simulink model "Twostage_TVC6DOF_sim"  (R2023b)
settings: Solver=VariableStepAuto  StartTime=0.0  StopTime=7  RelTol=1e-3
values from neighbouring files (symbols this model uses):
  g = 9.81    [TVC6DOF.m]
  ignition_delay_mc = ignition_delay_n+randn*ignition_delay_v    [TVC6DOF.m]
  Ix2_mc = Ix2_n+randn*Ix2_v    [TVC6DOF.m]
  Ix_mc = Ix_n+randn*Ix_v    [TVC6DOF.m]
  Iy2_mc = Iy2_n+randn*Iy2_v    [TVC6DOF.m]
  Iy_mc = Iy_n+randn*Iy_v    [TVC6DOF.m]
  Iz2_mc = Iz2_n+randn*Iz2_v    [TVC6DOF.m]
  Iz_mc = Iz_n+randn*Iz_v    [TVC6DOF.m]
  l2_mc = l2_n+randn*l2_v    [TVC6DOF.m]
  l_mc = l_n+randn*l_v    [TVC6DOF.m]
  m2_dry_mc = m2_dry_n+randn*m2_dry_v    [TVC6DOF.m]
  m_dry_mc = m_dry_n+randn*m_dry_v    [TVC6DOF.m]
  mis_y_mc = randn*mis_y_v    [TVC6DOF.m]
  mis_z_mc = randn*mis_z_v    [TVC6DOF.m]
  servo_delay_mc = servo_delay_n+randn*servo_delay_v    [TVC6DOF.m]
  twostage_delay_n = 1.5    [TVC6DOF.m]
undefined symbols (not defined in the file or in its folder): sigbuilder_block
settings Model: Creator=govindchari  LastModifiedBy=AISL
settings SolverCC: AlgebraicLoopSolver=TrustRegion
settings DebuggingCC: UnconnectedInputMsg=warning  UnconnectedOutputMsg=warning  UnconnectedLineMsg=warning
settings ModelReferenceCC: EnableRefExpFcnMdlSchedulingChecks=on
settings RTWCC: DLArmComputeVersion=19.05

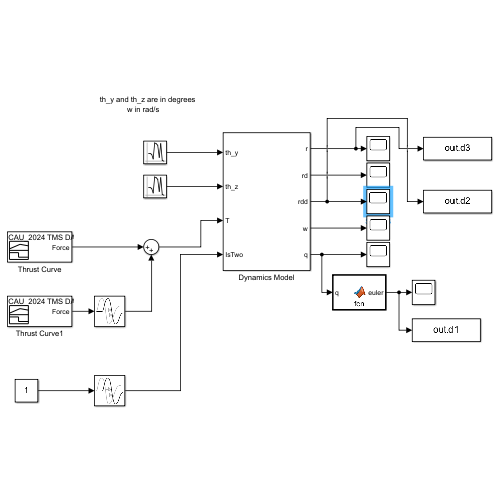
[thumbnail: Simulink's stored preview of the top-level diagram]
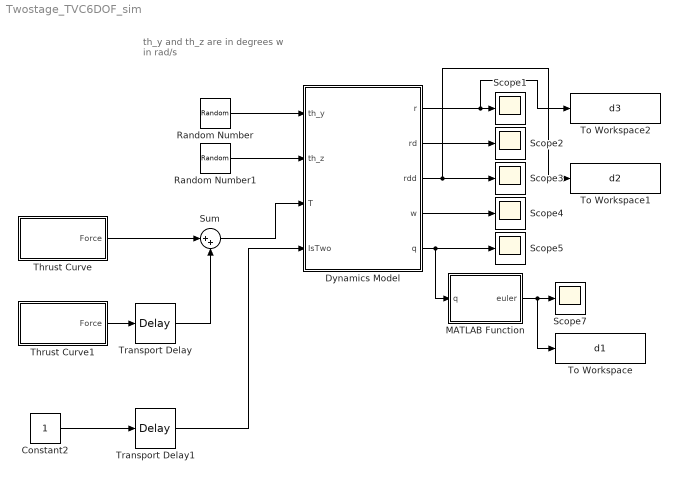
== system Twostage_TVC6DOF_sim ==
  note: th_y and th_z are in degrees
      |              w in rad/s
  Constant2 : Constant
  Dynamics Model : Subsystem
  MATLAB Function : MATLAB Function  TreatAsAtomicUnit=on
  Random Number : RandomNumber  Variance=0.1  SampleTime=0.001
  Random Number1 : RandomNumber  Variance=0.1  SampleTime=0.001
  Scope{1..5,7} (6 alike) : Scope
  Sum : Sum  Inputs=|++
  Thrust Curve : Subsystem  Tag=STV Subsys  LoadFcn=sigbuilder_block('load');  StartFcn=sigbuilder_block('start');  StopFcn=sigbuilder_block('stop');  ClipboardFcn=sigbuilder_block('clipboard');  mask(Sigbuilder block){tuvar=[0:10]}
      mask help: Simulink:masks:SigbuilderBlock_MD
      mask init:
      | if ~strcmp(get_param(bdroot(gcbh),'SimulationStatus'),'stopped') tuvar = sigbuilder_block('maskInit'); end
      settings: CopyFcn=sigbuilder_block('copy');  DeleteFcn=sigbuilder_block('delete');  ModelCloseFcn=sigbuilder_block('modelClose');  PreSaveFcn=sigbuilder_block('preSave');  PauseFcn=sigbuilder_block('pause');  ContinueFcn=sigbuilder_block('continue');  NameChangeFcn=sigbuilder_block('namechange');  OpenFcn=sigbuilder_block('open',[1201.5 112.5 712.5 317.25 ]);  CloseFcn=sigbuilder_block('close');
      mask Display: plot(0, 0, 100, 100,[2, 2, 32, 32, 2], [68, 8, 8, 68, 68],[32, 2], [38, 38], [32, 19, 2],[53, 60, 44], [32, 17, 17, 2],[16, 16, 31, 31]);txt = getActiveGroup(gcbh);text(2, 100, txt,'verticalAlignment', 'top');
  Thrust Curve1 : Subsystem  Tag=STV Subsys  LoadFcn=sigbuilder_block('load');  StartFcn=sigbuilder_block('start');  StopFcn=sigbuilder_block('stop');  ClipboardFcn=sigbuilder_block('clipboard');  mask(Sigbuilder block){tuvar=[0:10]}
      mask help: Simulink:masks:SigbuilderBlock_MD
      mask init:
      | if ~strcmp(get_param(bdroot(gcbh),'SimulationStatus'),'stopped') tuvar = sigbuilder_block('maskInit'); end
      settings: CopyFcn=sigbuilder_block('copy');  DeleteFcn=sigbuilder_block('delete');  ModelCloseFcn=sigbuilder_block('modelClose');  PreSaveFcn=sigbuilder_block('preSave');  PauseFcn=sigbuilder_block('pause');  ContinueFcn=sigbuilder_block('continue');  NameChangeFcn=sigbuilder_block('namechange');  OpenFcn=sigbuilder_block('open',[380.25 420 924.75 358.5 ]);  CloseFcn=sigbuilder_block('close');
      mask Display: plot(0, 0, 100, 100,[2, 2, 32, 32, 2], [68, 8, 8, 68, 68],[32, 2], [38, 38], [32, 19, 2],[53, 60, 44], [32, 17, 17, 2],[16, 16, 31, 31]);txt = getActiveGroup(gcbh);text(2, 100, txt,'verticalAlignment', 'top');
  To Workspace : ToWorkspace  VariableName=d1  SaveFormat=Timeseries  SampleTime=-1
  To Workspace1 : ToWorkspace  VariableName=d2  SaveFormat=Timeseries  SampleTime=-1
  To Workspace2 : ToWorkspace  VariableName=d3  SaveFormat=Timeseries  SampleTime=-1
  Transport Delay : TransportDelay  DelayTime=ignition_delay_mc+servo_delay_mc+twostage_delay_n
  Transport Delay1 : TransportDelay  DelayTime=servo_delay_mc+twostage_delay_n
  wires:
  Dynamics Model/1(r) -> To Workspace2/1, Scope1/1
  Dynamics Model/2(rd) -> Scope2/1
  Dynamics Model/5(q) -> MATLAB Function/1(q), Scope5/1
  Dynamics Model/4(w) -> Scope4/1
  Dynamics Model/3(rdd) -> Scope3/1, To Workspace1/1
  Random Number/1 -> Dynamics Model/1(th_y)
  Random Number1/1 -> Dynamics Model/2(th_z)
  Sum/1 -> Dynamics Model/3(T)
  Thrust Curve/1(Force) -> Sum/1
  Thrust Curve1/1(Force) -> Transport Delay/1
  Transport Delay/1 -> Sum/2
  Constant2/1 -> Transport Delay1/1
  Transport Delay1/1 -> Dynamics Model/4(IsTwo)
  MATLAB Function/1(euler) -> To Workspace/1, Scope7/1

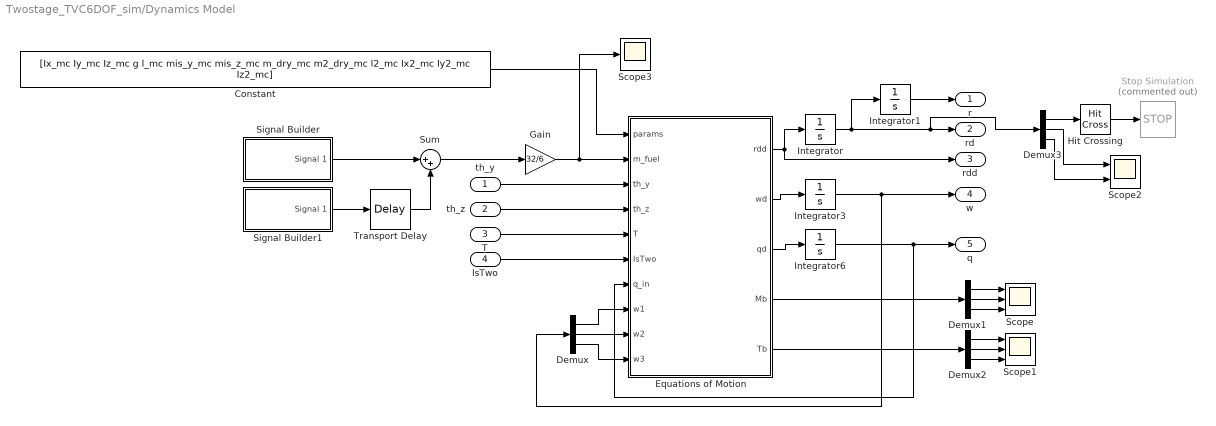
== system Twostage_TVC6DOF_sim/Dynamics Model ==
  th_y : Inport
  th_z : Inport  Port=2
  T : Inport  Port=3
  IsTwo : Inport  Port=4
  Constant : Constant  Value=[Ix_mc Iy_mc Iz_mc g l_mc mis_y_mc mis_z_mc m_dry_mc m2_dry_mc l2_mc Ix2_mc Iy2_mc Iz2_mc]
  Demux{,1..3} (4 alike) : Demux  Outputs=3
  Equations of Motion : MATLAB Function  TreatAsAtomicUnit=on
  Gain : Gain  Gain=32/6
  Hit Crossing : HitCross  HitCrossingOffset=0.01  HitCrossingDirection=falling
  Integrator : Integrator  InitialCondition=[0 0 0]
  Integrator1 : Integrator  InitialCondition=[0 0 0]
  Integrator3 : Integrator  InitialCondition=[0 0 0]
  Integrator6 : Integrator  InitialCondition=[1 0 0 0]
  Scope : Scope  NumInputPorts=3
  Scope1 : Scope  NumInputPorts=3
  Scope2 : Scope  NumInputPorts=2
  Scope3 : Scope
  Signal Builder : Subsystem  Tag=STV Subsys  LoadFcn=sigbuilder_block('load');  StartFcn=sigbuilder_block('start');  StopFcn=sigbuilder_block('stop');  ClipboardFcn=sigbuilder_block('clipboard');  mask(Sigbuilder block){tuvar=[0:10]}
      mask help: Simulink:masks:SigbuilderBlock_MD
      mask init:
      | if ~strcmp(get_param(bdroot(gcbh),'SimulationStatus'),'stopped') tuvar = sigbuilder_block('maskInit'); end
      settings: CopyFcn=sigbuilder_block('copy');  DeleteFcn=sigbuilder_block('delete');  ModelCloseFcn=sigbuilder_block('modelClose');  PreSaveFcn=sigbuilder_block('preSave');  PauseFcn=sigbuilder_block('pause');  ContinueFcn=sigbuilder_block('continue');  NameChangeFcn=sigbuilder_block('namechange');  OpenFcn=sigbuilder_block('open',[1949.25 96 550.5 400.5 ]);  CloseFcn=sigbuilder_block('close');
      mask Display: plot(0, 0, 100, 100,[2, 2, 32, 32, 2], [68, 8, 8, 68, 68],[32, 2], [38, 38], [32, 19, 2],[53, 60, 44], [32, 17, 17, 2],[16, 16, 31, 31]);txt = getActiveGroup(gcbh);text(2, 100, txt,'verticalAlignment', 'top');
  Signal Builder1 : Subsystem  Tag=STV Subsys  LoadFcn=sigbuilder_block('load');  StartFcn=sigbuilder_block('start');  StopFcn=sigbuilder_block('stop');  ClipboardFcn=sigbuilder_block('clipboard');  mask(Sigbuilder block){tuvar=[0:10]}
      mask help: Simulink:masks:SigbuilderBlock_MD
      mask init:
      | if ~strcmp(get_param(bdroot(gcbh),'SimulationStatus'),'stopped') tuvar = sigbuilder_block('maskInit'); end
      settings: CopyFcn=sigbuilder_block('copy');  DeleteFcn=sigbuilder_block('delete');  ModelCloseFcn=sigbuilder_block('modelClose');  PreSaveFcn=sigbuilder_block('preSave');  PauseFcn=sigbuilder_block('pause');  ContinueFcn=sigbuilder_block('continue');  NameChangeFcn=sigbuilder_block('namechange');  OpenFcn=sigbuilder_block('open',[1949.25 96 550.5 400.5 ]);  CloseFcn=sigbuilder_block('close');
      mask Display: plot(0, 0, 100, 100,[2, 2, 32, 32, 2], [68, 8, 8, 68, 68],[32, 2], [38, 38], [32, 19, 2],[53, 60, 44], [32, 17, 17, 2],[16, 16, 31, 31]);txt = getActiveGroup(gcbh);text(2, 100, txt,'verticalAlignment', 'top');
  Stop Simulation : Stop  Commented=on
  Sum : Sum  Inputs=|++
  Transport Delay : TransportDelay  DelayTime=ignition_delay_mc+servo_delay_mc+twostage_delay_n  InitialOutput=60
  r : Outport
  rd : Outport  Port=2
  rdd : Outport  Port=3
  w : Outport  Port=4
  q : Outport  Port=5
  wires:
  Constant/1 -> Equations of Motion/1(params)
  Equations of Motion/3(qd) -> Integrator6/1
  Equations of Motion/2(wd) -> Integrator3/1
  Equations of Motion/1(rdd) -> Integrator/1, rdd/1
  T/1 -> Equations of Motion/5(T)
  Integrator/1 -> Integrator1/1, Demux3/1, rd/1
  Integrator1/1 -> r/1
  Demux/1 -> Equations of Motion/8(w1)
  Demux/2 -> Equations of Motion/9(w2)
  Demux/3 -> Equations of Motion/10(w3)
  Integrator6/1 -> Equations of Motion/7(q_in), q/1
  Integrator3/1 -> Demux/1, w/1
  Equations of Motion/4(Mb) -> Demux1/1
  Equations of Motion/5(Tb) -> Demux2/1
  Demux1/1 -> Scope/1
  Demux1/2 -> Scope/2
  Demux1/3 -> Scope/3
  Demux2/1 -> Scope1/1
  Demux2/2 -> Scope1/2
  Demux2/3 -> Scope1/3
  Demux3/1 -> Hit Crossing/1
  Hit Crossing/1 -> Stop Simulation/1
  Demux3/2 -> Scope2/1
  Demux3/3 -> Scope2/2
  th_z/1 -> Equations of Motion/4(th_z)
  th_y/1 -> Equations of Motion/3(th_y)
  Gain/1 -> Scope3/1, Equations of Motion/2(m_fuel)
  IsTwo/1 -> Equations of Motion/6(IsTwo)
  Signal Builder/1(Signal 1) -> Sum/1
  Sum/1 -> Gain/1
  Signal Builder1/1(Signal 1) -> Transport Delay/1
  Transport Delay/1 -> Sum/2

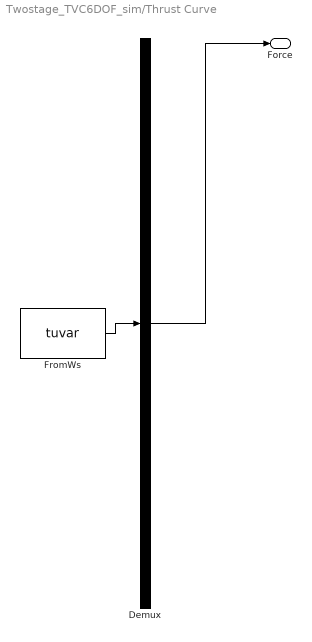
== system Twostage_TVC6DOF_sim/Thrust Curve ==
  Demux : Demux  Tag=STV Demux  Outputs=1
      settings: DisplayOption=none
  FromWs : FromWorkspace  Tag=STV FromWs  VariableName=tuvar
      SigBuilderData=|
      | common.afterFinalStr = 'Extrapolate'
      | common.sampleTime = 0
      | dataSet.timeRange = [0 7]
      | dataSet.name = 'CAU_2024 TMS DATA_0525'
      | sbobj.Groups.Name = 'CAU_2024 TMS DATA_0525'
      | sbobj.Groups.Signals.Name = 'Force'
      | sbobj.Groups.Signals.XData = [0 0.06 0.13 0.2 0.27 0.34 0.41 0.47 0.54 0.61 0.68 0.75 0.82 0.88 0.95 1.02 1.09 1.16 1.23 1.3 1.36 1.43 1.5 1.56 1.63 1.7 1.77 1.84 1.9 1.97 2.04 2.11 2.17 2.24 2.31 2.38 2.44 2.51 2.58 7]
      | sbobj.Groups.Signals.YData = [20.593965 10.591182 23.339827 42.6589275 69.7252815 112.4822755 170.047311 259.7781585 451.890432 466.3340375 466.432104 467.412769 479.371316 469.346269 340.094622 265.6621485 130.9187775 44.8163905 20.986231 10.4931155 2.2555295 1.569064 0.0980665 0 1.4709975 0.2941995 0.784532 0.196133 0 0 0.392266 0 1.6671305 1.176798 0 1.2748645 0.2941995 0 1.372931 1.372931]
      | sbobj.Groups.TimeRange = [0 7]
  Force : Outport  Tag=STV Outport
  wires:
  Demux/1 -> Force/1
  FromWs/1 -> Demux/1

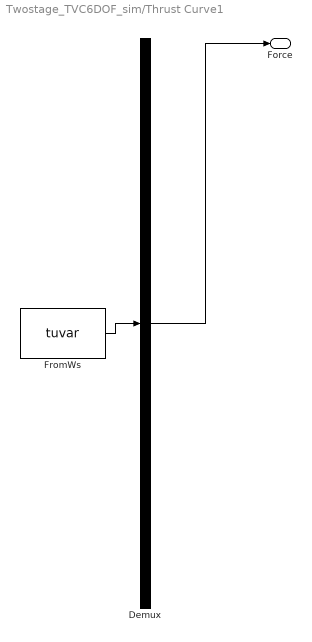
== system Twostage_TVC6DOF_sim/Thrust Curve1 ==
  Demux : Demux  Tag=STV Demux  Outputs=1
      settings: DisplayOption=none
  FromWs : FromWorkspace  Tag=STV FromWs  VariableName=tuvar
      SigBuilderData=|
      | common.afterFinalStr = 'Extrapolate'
      | common.sampleTime = 0
      | dataSet(1).timeRange = [0 2.58]
      | dataSet(1).name = 'CAU_2024 TMS DATA_0525'
      | dataSet(2).timeRange = [0 7]
      | dataSet(2).name = 'CAU_2024 TMS DATA_1'
      | dataSet(3).timeRange = [0 7]
      | dataSet(3).name = 'CAU_2024 TMS DATA_2'
      | sbobj.Groups(1).Name = 'CAU_2024 TMS DATA_0525'
      | sbobj.Groups(1).Signals.Name = 'Force'
      | sbobj.Groups(1).Signals.XData = [0 0.06 0.13 0.2 0.27 0.34 0.41 0.47 0.54 0.61 0.68 0.75 0.82 0.88 0.95 1.02 1.09 1.16 1.23 1.3 1.36 1.43 1.5 1.56 1.63 1.7 1.77 1.84 1.9 1.97 2.04 2.11 2.17 2.24 2.31 2.38 2.44 2.51 2.58]
      | sbobj.Groups(1).Signals.YData = [20.593965 10.591182 23.339827 42.6589275 69.7252815 112.4822755 170.047311 259.7781585 451.890432 466.3340375 466.432104 467.412769 479.371316 469.346269 340.094622 265.6621485 130.9187775 44.8163905 20.986231 10.4931155 2.2555295 1.569064 0.0980665 0 1.4709975 0.2941995 0.784532 0.196133 0 0 0.392266 0 1.6671305 1.176798 0 1.2748645 0.2941995 0 1.372931]
      | sbobj.Groups(1).TimeRange = [0 2.58]
      | sbobj.Groups(2).Name = 'CAU_2024 TMS DATA_1'
      | sbobj.Groups(2).Signals.Name = 'Force'
      | sbobj.Groups(2).Signals.XData = [0 0.06 0.13 0.2 0.27 0.34 0.41 0.47 0.54 0.61 0.68 0.75 0.82 0.88 0.95 1.02 1.09 1.16 1.23 1.3 1.36 1.43 1.5 1.56 1.63 1.7 1.77 1.84 1.9 1.97 2.04 2.11 2.17 2.24 2.31 2.38 2.44 2.51 2.58 7]
      | sbobj.Groups(2).Signals.YData = [20.593965 10.591182 23.339827 42.6589275 69.7252815 112.4822755 170.047311 259.7781585 451.890432 466.3340375 466.432104 467.412769 479.371316 469.346269 340.094622 265.6621485 130.9187775 44.8163905 20.986231 10.4931155 2.2555295 1.569064 0.0980665 0 1.4709975 0.2941995 0.784532 0.196133 0 0 0.392266 0 1.6671305 1.176798 0 1.2748645 0.2941995 0 1.372931 1.372931]
      | sbobj.Groups(2).TimeRange = [0 7]
      | sbobj.Groups(3).Name = 'CAU_2024 TMS DATA_2'
      | sbobj.Groups(3).Signals.Name = 'Force'
      | sbobj.Groups(3).Signals.XData = [0 2 2.07 2.14 2.21 2.27 2.34 2.41 2.48 2.54 2.61 2.68 2.75 2.82 2.89 2.95 3.02 3.09 3.16 3.23 3.3 3.36 3.43 3.5 3.57 3.64 3.71 3.78 3.84 3.91 3.98 4.04 4.11 4.18 4.25 4.32 4.38 4.45 4.52 4.59 4.65 4.72 4.79 4.86 4.92 4.99 5.06 7]
      | sbobj.Groups(3).Signals.YData = [0 0 0 0 0 0.392266 0 0.392266 20.593965 10.591182 23.339827 42.6589275 69.7252815 112.4822755 170.047311 259.7781585 451.890432 466.3340375 466.432104 467.412769 479.371316 469.346269 340.094622 265.6621485 130.9187775 44.8163905 20.986231 10.4931155 2.2555295 1.569064 0.0980665 0 1.4709975 0.2941995 0.784532 0.196133 0 0 0.392266 0 1.6671305 1.176798 0 1.2748645 0.2941995 0 1.372931 1.372931]
      | sbobj.Groups(3).TimeRange = [0 7]
  Force : Outport  Tag=STV Outport
  wires:
  Demux/1 -> Force/1
  FromWs/1 -> Demux/1

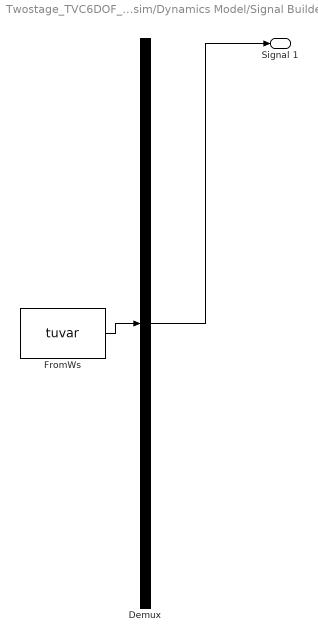
== system Twostage_TVC6DOF_sim/Dynamics Model/Signal Builder ==
  Demux : Demux  Tag=STV Demux  Outputs=1
      settings: DisplayOption=none
  FromWs : FromWorkspace  Tag=STV FromWs  VariableName=tuvar
      SigBuilderData=|
      | common.afterFinalStr = 'Extrapolate'
      | common.sampleTime = 0
      | dataSet.timeRange = [0 10]
      | dataSet.name = 'Group 1'
      | sbobj.Groups.Name = 'Group 1'
      | sbobj.Groups.Signals.Name = 'Signal 1'
      | sbobj.Groups.Signals.XData = [0 0.148 0.228 0.294 0.419 0.477 0.52 0.593 0.628 0.755 0.837 1 1.123 1.152 1.163 1.286 1.455 1.61 1.694 1.71 1.72 1.75 3.404 3.404 3.45 9.8 10]
      | sbobj.Groups.Signals.YData = [60 59.3164 58.3541 57.2108 54.0771 52.3818 51.2397 49.4767 47.3744 43.9685 40.4849 37.3989 33.5 32.9674 32.026 27.8823 24.0514 19.5 14.8632 10.4455 4.68731 0.51289 0.215344 0.0947253 0 0 0]
  Signal 1 : Outport  Tag=STV Outport
  wires:
  Demux/1 -> Signal 1/1
  FromWs/1 -> Demux/1

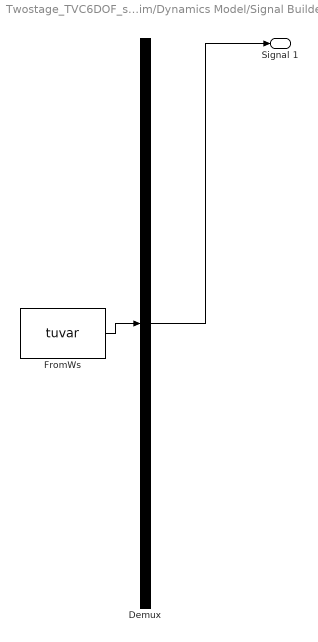
== system Twostage_TVC6DOF_sim/Dynamics Model/Signal Builder1 ==
  Demux : Demux  Tag=STV Demux  Outputs=1
      settings: DisplayOption=none
  FromWs : FromWorkspace  Tag=STV FromWs  VariableName=tuvar
      SigBuilderData=|
      | common.afterFinalStr = 'Extrapolate'
      | common.sampleTime = 0
      | dataSet.timeRange = [0 10]
      | dataSet.name = 'Group 1'
      | sbobj.Groups.Name = 'Group 1'
      | sbobj.Groups.Signals.Name = 'Signal 1'
      | sbobj.Groups.Signals.XData = [0 0.148 0.228 0.294 0.419 0.477 0.52 0.593 0.628 0.755 0.837 1 1.123 1.152 1.163 1.286 1.455 1.61 1.694 1.71 1.72 1.75 3.404 3.404 3.45 9.8 10]
      | sbobj.Groups.Signals.YData = [60 59.3164 58.3541 57.2108 54.0771 52.3818 51.2397 49.4767 47.3744 43.9685 40.4849 37.3989 33.5 32.9674 32.026 27.8823 24.0514 19.5 14.8632 10.4455 4.68731 0.51289 0.215344 0.0947253 0 0 0]
  Signal 1 : Outport  Tag=STV Outport
  wires:
  Demux/1 -> Signal 1/1
  FromWs/1 -> Demux/1

== matlab function Twostage_TVC6DOF_sim/MATLAB Function ==
  data: q input; euler output
function euler = fcn(q)
euler=[1,1,1];
euler = quat2eul(q');

== matlab function Twostage_TVC6DOF_sim/Dynamics Model/Equations of Motion ==
  data: params input; m_fuel input; th_y input; rdd output; th_z input; T input; IsTwo input; q_in input; wd output; qd output; w1 input; w2 input; w3 input; Mb output; Tb output
function [rdd,wd,qd,Mb,Tb] = EOM(params,m_fuel,th_y,th_z,T,IsTwo, q_in,w1,w2,w3)
Ix=params(1);
Iy=params(2);
Iz=params(3);
g=params(4);
l=params(5);
mis_y=params(6);
mis_z=params(7);
m_dry=params(8);
m2_dry=params(9);
l2=params(10);
Ix2=params(11);
Iy2=params(12);
Iz2=params(13);

if(IsTwo==0)
    m=m_dry+m_fuel/1000;
else
    m=m2_dry+m_fuel/1000;
    Ix=Ix2;
    Iy=Iy2;
    Iz=Iz2;
end
wx=w1;
wy=w2;
wz=w3;

if size(q_in)==1
    q_in=[1;0;0;0];
end
%gCb=[cosd(th_z) sind(th_z) 0;-sind(th_z) cosd(th_z) 0;0 0 1]*[cosd(th_y) 0 -sind(th_y);0 1 0;sind(th_y) 0 cosd(th_y)];
Tb=[T;0;0];
if(IsTwo==0)
    r=[-l;mis_y;mis_z];
else
    r=[-l2;mis_y;mis_z];
end

Mb=cross(r,Tb);
Ti=hamilton(hamilton(q_in,[0;Tb]),conjugate(q_in));

xdd=Ti(2)/m-g;
ydd=Ti(3)/m+th_y;
zdd=Ti(4)/m+th_z;

rdd=[xdd;ydd;zdd];

wxd=(1/Ix)*(Mb(1)+(Iy-Iz)*wy*wz);
wyd=(1/Iy)*(Mb(2)+(Iz-Ix)*wx*wz);
wzd=(1/Iz)*(Mb(3)+(Ix-Iy)*wx*wy);

wd=[wxd;wyd;wzd];

qd=0.5*hamilton(q_in,[0;wx;wy;wz]);
    function product=hamilton(q,r)
        product=[r(1)*q(1)-r(2)*q(2)-r(3)*q(3)-r(4)*q(4);
                 r(1)*q(2)+r(2)*q(1)-r(3)*q(4)+r(4)*q(3);
                 r(1)*q(3)+r(2)*q(4)+r(3)*q(1)-r(4)*q(2);
                 r(1)*q(4)-r(2)*q(3)+r(3)*q(2)+r(4)*q(1)];
    end

    function q_star=conjugate(q)
        q_star=[q(1);-q(2);-q(3);-q(4)];
    end
end
